simulink model "f14autopilot"  (Simulink 7.6)
settings: Solver=ode45  SolverMode=SingleTasking  StartTime=0.0  StopTime=10.0  RelTol=1e-3  AbsTol=1e-6
PreLoadFcn:
  | load f14_digital_data.mat
values from neighbouring files (symbols this model uses):
  Ka = 0.677    [f14_digital_data.mat]    (also in f14dat_digital.m)
  Kf = -1.746    [f14_digital_data.mat]    (also in f14dat_digital.m)
  Ki = -3.864    [f14_digital_data.mat]    (also in f14dat_digital.m)
  Kq = 0.8156    [f14_digital_data.mat]    (also in f14dat_digital.m)
  Tal = 0.3959    [f14_digital_data.mat]    (also in f14dat_digital.m)
  Ts = 0.1    [f14_digital_data.mat]    (also in f14dat_digital.m)
  W1 = 2.971    [f14_digital_data.mat]    (also in f14dat_digital.m)
  W2 = 4.144    [f14_digital_data.mat]    (also in f14dat_digital.m)
Description:
  | Analog autopilot design baseline for F-14 control design demonstration
settings Model: Creator=The MathWorks Inc.  ExtModeTrigMode=oneshot  ExtModeArmWhenConnect=off  ExtModeAutoUpdateStatusClock=off  BufferReuse=off
settings DataIOCC: InitialState=[]  LimitDataPoints=off  LoadInitialState=on  SignalLoggingName=logsOut
settings OptimizationCC: BooleanDataType=off  InlineParams=on  InlineInvariantSignals=on  BufferReuse=off  InitFltsAndDblsToZero=on
settings DebuggingCC: SaveWithParameterizedLinksMsg=none  CheckExecutionContextPreStartOutputMsg=on  CheckExecutionContextRuntimeOutputMsg=on  SignalResolutionControl=TryResolveAllWithWarning  SolverPrmCheckMsg=none  MultiTaskDSMMsg=warning  MultiTaskCondExecSysMsg=none  IntegerOverflowMsg=none
settings RTWCC: TemplateMakefile=grt_vc.tmf  IncludeERTFirstTime=on
settings GRTTargetCC: TargetFcnLib=ansi_tfl_tmw.mat

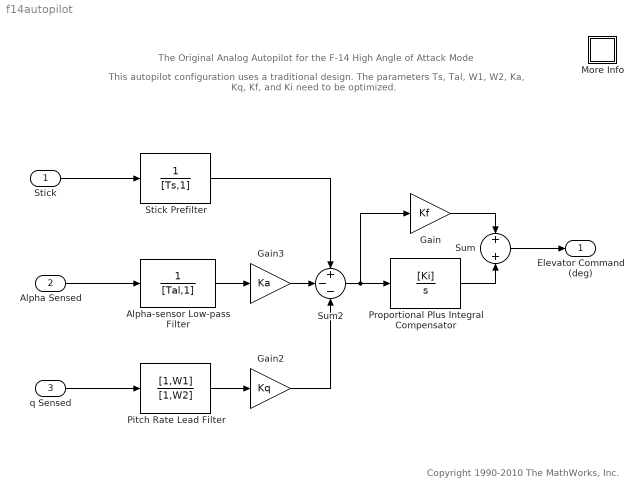
== system f14autopilot ==
  note: The Original Analog Autopilot for the F-14 High Angle of Attack Mode
  note: This autopilot configuration uses a traditional design.
      | The parameters Ts, Tal, W1, W2, Ka, Kq, Kf, and Ki need to be optimized.
  note: Copyright 1990-2010 The MathWorks, Inc.
  Stick : Inport  PortDimensions=1
  Alpha Sensed : Inport  Port=2  PortDimensions=1
  q Sensed : Inport  Port=3  PortDimensions=1
  Alpha-sensor Low-pass Filter : TransferFcn  Denominator=[Tal,1]
  Gain : Gain  Gain=Kf  SaturateOnIntegerOverflow=on  OutDataTypeStr=Inherit: Same as input  ParamDataTypeStr=Inherit: Same as input
  Gain2 : Gain  Gain=Kq  SaturateOnIntegerOverflow=on  OutDataTypeStr=Inherit: Same as input  ParamDataTypeStr=Inherit: Same as input
  Gain3 : Gain  Gain=Ka  SaturateOnIntegerOverflow=on  OutDataTypeStr=Inherit: Same as input  ParamDataTypeStr=Inherit: Same as input
  More Info : Subsystem
      settings: OpenFcn=showdemo('sldemo_f14dig_script')
      mask Display: disp('?')
  Pitch Rate Lead Filter : TransferFcn  Numerator=[1,W1]  Denominator=[1,W2]
  Proportional Plus Integral Compensator : TransferFcn  Numerator=[Ki]  Denominator=[1,0]
  Stick Prefilter : TransferFcn  Denominator=[Ts,1]
  Sum : Sum  Inputs=2  SaturateOnIntegerOverflow=on  InputSameDT=on  OutDataTypeStr=Inherit: Same as first input
  Sum2 : Sum  Inputs=+--  SaturateOnIntegerOverflow=on  InputSameDT=on  OutDataTypeStr=Inherit: Same as first input
  Elevator Command (deg) : Outport  InitialOutput=0
  wires:
  Stick Prefilter/1 -> Sum2/1
  Pitch Rate Lead Filter/1 -> Gain2/1
  Alpha-sensor Low-pass Filter/1 -> Gain3/1
  Gain3/1 -> Sum2/2
  Gain2/1 -> Sum2/3
  Stick/1 -> Stick Prefilter/1
  Sum2/1 -> Proportional Plus Integral Compensator/1, Gain/1
  Gain/1 -> Sum/1
  Alpha Sensed/1 -> Alpha-sensor Low-pass Filter/1
  q Sensed/1 -> Pitch Rate Lead Filter/1
  Sum/1 -> Elevator Command (deg)/1
  Proportional Plus Integral Compensator/1 -> Sum/2

== system f14autopilot/More Info ==
